simulink model "multiloop"  (R2017b)
settings: Solver=ode4  StartTime=0.0  StopTime=15  FixedStep=1e-3  RelTol=1e-3
values from neighbouring files (symbols this model uses):
  K11 = 0.97    [T3_Master_MultiLoopControl_ejemplo.m]
  K12 = -0.3    [T3_Master_MultiLoopControl_ejemplo.m]
  K13 = 1.1    [T3_Master_MultiLoopControl_ejemplo.m]
  K21 = 1    [T3_Master_MultiLoopControl_ejemplo.m]
  K22 = -0.8    [T3_Master_MultiLoopControl_ejemplo.m]
  K23 = 0.91    [T3_Master_MultiLoopControl_ejemplo.m]
  K31 = 0.5    [T3_Master_MultiLoopControl_ejemplo.m]
  K32 = -0.3    [T3_Master_MultiLoopControl_ejemplo.m]
  K33 = 0.55    [T3_Master_MultiLoopControl_ejemplo.m]
  Ki_1 = wn_mod^2/b11    (= 2.8224742268)    [T3_Master_MultiLoopControl_ejemplo.m]
  Ki_2 = wn_mod^2/b22    (= -3.9355875)    [T3_Master_MultiLoopControl_ejemplo.m]
  Ki_3 = wn_mod^2/b33    (= 4.48003636364)    [T3_Master_MultiLoopControl_ejemplo.m]
  Kp_1 = (2*xi_mod*wn_mod-a11)/b11    (= 3.79381443299)    [T3_Master_MultiLoopControl_ejemplo.m]
  Kp_2 = (2*xi_mod*wn_mod-a22)/b22    (= -5.4775)    [T3_Master_MultiLoopControl_ejemplo.m]
  Kp_3 = (2*xi_mod*wn_mod-a33)/b33    (= 5.84)    [T3_Master_MultiLoopControl_ejemplo.m]
  tau1 = 2    [T3_Master_MultiLoopControl_ejemplo.m]
  tau2 = 2.3    [T3_Master_MultiLoopControl_ejemplo.m]
  tau3 = 1.8    [T3_Master_MultiLoopControl_ejemplo.m]
settings Model: Creator=pablo  LastModifiedBy=pablo

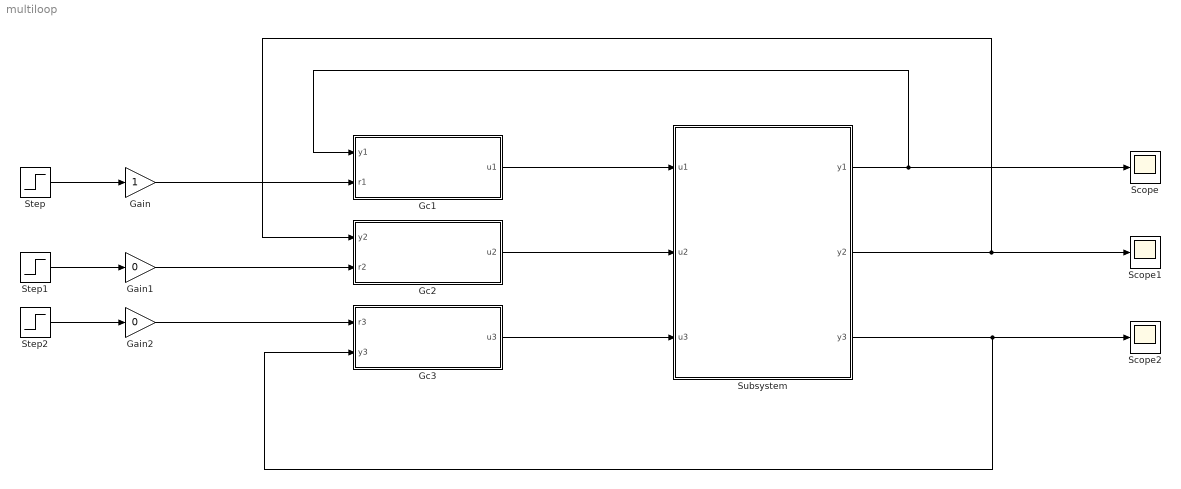
== system multiloop ==
  Gain : Gain
  Gain1 : Gain  Gain=0
  Gain2 : Gain  Gain=0
  Gc1 : Subsystem
  Gc2 : Subsystem
  Gc3 : Subsystem
  Scope : Scope
  Scope1 : Scope
  Scope2 : Scope
  Step : Step  SampleTime=0
  Step1 : Step  SampleTime=0
  Step2 : Step  SampleTime=0
  Subsystem : Subsystem
  wires:
  Step/1 -> Gain/1
  Step1/1 -> Gain1/1
  Step2/1 -> Gain2/1
  Subsystem/1(y1) -> Gc1/1(y1), Scope/1
  Subsystem/2(y2) -> Gc2/1(y2), Scope1/1
  Subsystem/3(y3) -> Gc3/2(y3), Scope2/1
  Gain/1 -> Gc1/2(r1)
  Gc1/1(u1) -> Subsystem/1(u1)
  Gc2/1("u2 ") -> Subsystem/2(u2)
  Gain1/1 -> Gc2/2("r2 ")
  Gain2/1 -> Gc3/1("r3 ")
  Gc3/1("u3 ") -> Subsystem/3(u3)

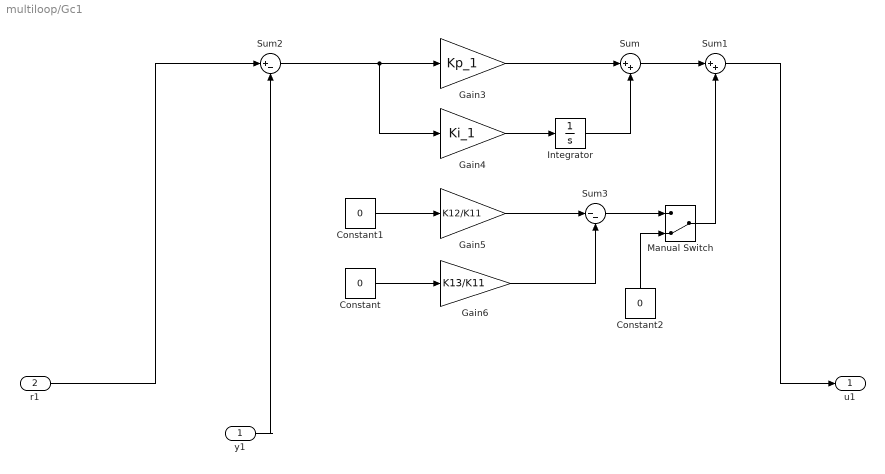
== system multiloop/Gc1 ==
  y1 : Inport
  r1 : Inport  Port=2
  Constant : Constant  Value=0
  Constant1 : Constant  Value=0
  Constant2 : Constant  Value=0
  Gain3 : Gain  Gain=Kp_1
  Gain4 : Gain  Gain=Ki_1
  Gain5 : Gain  Gain=K12/K11
  Gain6 : Gain  Gain=K13/K11
  Integrator : Integrator
  Manual Switch : ManualSwitch  CurrentSetting=0
  Sum : Sum  Inputs=|++
  Sum1 : Sum  Inputs=|++
  Sum2 : Sum  Inputs=|+-
  Sum3 : Sum  Inputs=|--
  u1 : Outport
  wires:
  Gain3/1 -> Sum/1
  Gain5/1 -> Sum3/1
  Gain4/1 -> Integrator/1
  Constant/1 -> Gain6/1
  Sum2/1 -> Gain4/1, Gain3/1
  Integrator/1 -> Sum/2
  Gain6/1 -> Sum3/2
  Sum/1 -> Sum1/1
  Sum1/1 -> u1/1
  y1/1 -> Sum2/2
  Constant1/1 -> Gain5/1
  r1/1 -> Sum2/1
  Constant2/1 -> Manual Switch/2
  Sum3/1 -> Manual Switch/1
  Manual Switch/1 -> Sum1/2

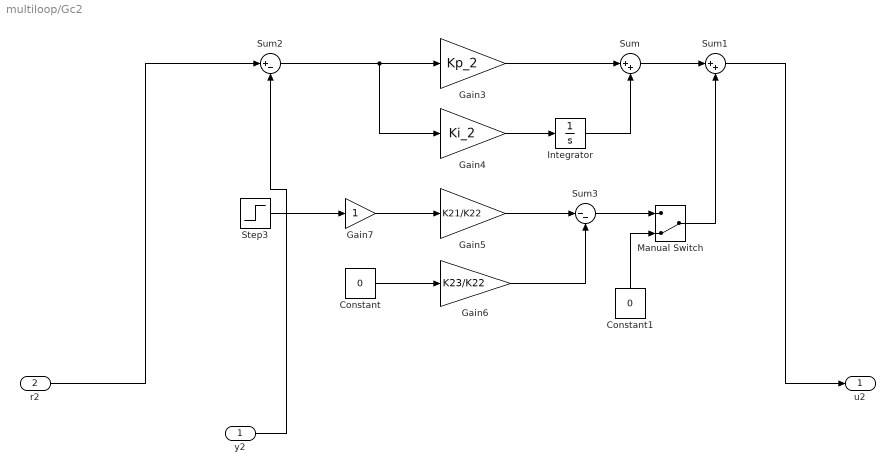
== system multiloop/Gc2 ==
  y2 : Inport
  "r2 " : Inport  Port=2
  Constant : Constant  Value=0
  Constant1 : Constant  Value=0
  Gain3 : Gain  Gain=Kp_2
  Gain4 : Gain  Gain=Ki_2
  Gain5 : Gain  Gain=K21/K22
  Gain6 : Gain  Gain=K23/K22
  Gain7 : Gain
  Integrator : Integrator
  Manual Switch : ManualSwitch  CurrentSetting=0
  Step3 : Step  SampleTime=0
  Sum : Sum  Inputs=|++
  Sum1 : Sum  Inputs=|++
  Sum2 : Sum  Inputs=|+-
  Sum3 : Sum  Inputs=|--
  "u2 " : Outport
  wires:
  Gain6/1 -> Sum3/2
  Integrator/1 -> Sum/2
  Sum/1 -> Sum1/1
  Sum2/1 -> Gain4/1, Gain3/1
  y2/1 -> Sum2/2
  Gain5/1 -> Sum3/1
  Step3/1 -> Gain7/1
  "r2 "/1 -> Sum2/1
  Sum1/1 -> "u2 "/1
  Gain3/1 -> Sum/1
  Gain7/1 -> Gain5/1
  Gain4/1 -> Integrator/1
  Constant/1 -> Gain6/1
  Sum3/1 -> Manual Switch/1
  Manual Switch/1 -> Sum1/2
  Constant1/1 -> Manual Switch/2

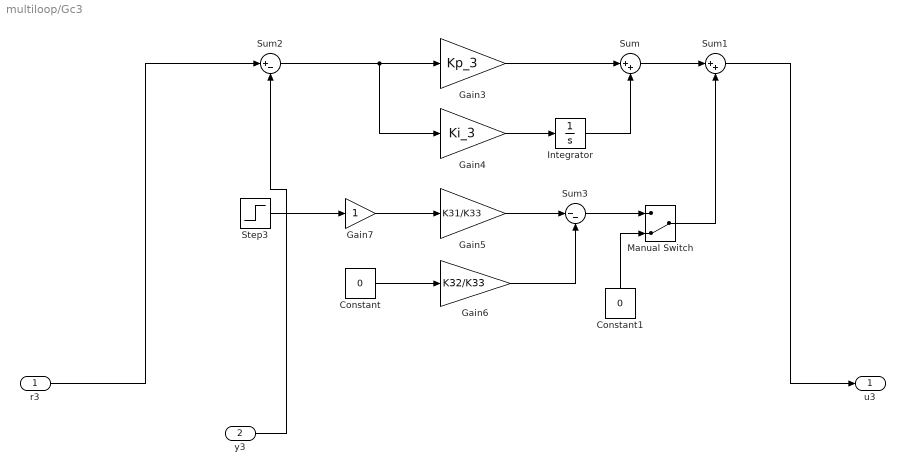
== system multiloop/Gc3 ==
  "r3 " : Inport
  y3 : Inport  Port=2
  Constant : Constant  Value=0
  Constant1 : Constant  Value=0
  Gain3 : Gain  Gain=Kp_3
  Gain4 : Gain  Gain=Ki_3
  Gain5 : Gain  Gain=K31/K33
  Gain6 : Gain  Gain=K32/K33
  Gain7 : Gain
  Integrator : Integrator
  Manual Switch : ManualSwitch  CurrentSetting=0
  Step3 : Step  SampleTime=0
  Sum : Sum  Inputs=|++
  Sum1 : Sum  Inputs=|++
  Sum2 : Sum  Inputs=|+-
  Sum3 : Sum  Inputs=|--
  "u3 " : Outport
  wires:
  Gain7/1 -> Gain5/1
  "r3 "/1 -> Sum2/1
  Sum/1 -> Sum1/1
  Step3/1 -> Gain7/1
  Gain6/1 -> Sum3/2
  Gain3/1 -> Sum/1
  Sum1/1 -> "u3 "/1
  Gain5/1 -> Sum3/1
  Gain4/1 -> Integrator/1
  Integrator/1 -> Sum/2
  y3/1 -> Sum2/2
  Sum2/1 -> Gain4/1, Gain3/1
  Constant/1 -> Gain6/1
  Constant1/1 -> Manual Switch/2
  Sum3/1 -> Manual Switch/1
  Manual Switch/1 -> Sum1/2

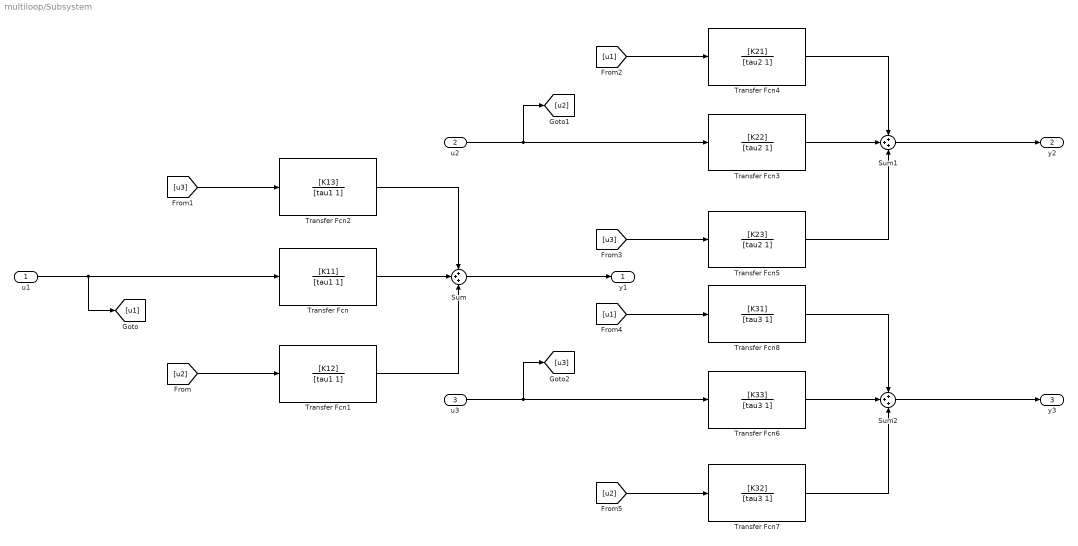
== system multiloop/Subsystem ==
  u1 : Inport
  u2 : Inport  Port=2
  u3 : Inport  Port=3
  Sum : Sum  Inputs=+++
  Sum1 : Sum  Inputs=+++
  Sum2 : Sum  Inputs=+++
  Transfer Fcn : TransferFcn  Numerator=[K11]  Denominator=[tau1 1]
  Transfer Fcn1 : TransferFcn  Numerator=[K12]  Denominator=[tau1 1]
  Transfer Fcn2 : TransferFcn  Numerator=[K13]  Denominator=[tau1 1]
  Transfer Fcn3 : TransferFcn  Numerator=[K22]  Denominator=[tau2 1]
  Transfer Fcn4 : TransferFcn  Numerator=[K21]  Denominator=[tau2 1]
  Transfer Fcn5 : TransferFcn  Numerator=[K23]  Denominator=[tau2 1]
  Transfer Fcn6 : TransferFcn  Numerator=[K33]  Denominator=[tau3 1]
  Transfer Fcn7 : TransferFcn  Numerator=[K32]  Denominator=[tau3 1]
  Transfer Fcn8 : TransferFcn  Numerator=[K31]  Denominator=[tau3 1]
  y1 : Outport
  y2 : Outport  Port=2
  y3 : Outport  Port=3
  wires:
  [u2] -> Transfer Fcn7/1
  Transfer Fcn1/1 -> Sum/3
  Transfer Fcn8/1 -> Sum2/1
  Transfer Fcn5/1 -> Sum1/3
  u2/1 -> [u2], Transfer Fcn3/1
  Transfer Fcn/1 -> Sum/2
  Transfer Fcn2/1 -> Sum/1
  Transfer Fcn4/1 -> Sum1/1
  [u3] -> Transfer Fcn5/1
  u1/1 -> [u1], Transfer Fcn/1
  Transfer Fcn3/1 -> Sum1/2
  [u3] -> Transfer Fcn2/1
  Sum/1 -> y1/1
  Sum1/1 -> y2/1
  [u1] -> Transfer Fcn8/1
  Transfer Fcn7/1 -> Sum2/3
  Sum2/1 -> y3/1
  [u2] -> Transfer Fcn1/1
  [u1] -> Transfer Fcn4/1
  Transfer Fcn6/1 -> Sum2/2
  u3/1 -> [u3], Transfer Fcn6/1
